simulink model "sendRecieve"  (R2016a)
settings: Solver=VariableStepAuto  StartTime=0.0  StopTime=10.0  RelTol=1e-3
libraries: instrumentlib x3
settings Model: Creator=Ori  LastModifiedBy=Ori

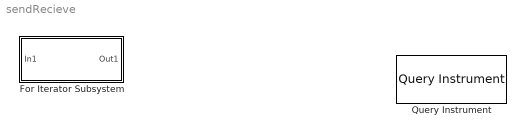
== system sendRecieve ==
  For Iterator Subsystem : Subsystem  TreatAsAtomicUnit=on
  Query Instrument : instrumentlib/Query Instrument  sampleTime=1  isWorkspaceObject=off  timeout=10  inputBufferSize=512  protocol=Serial  serialPort=COM1  baudRate=9600  gpibVendor=Advantech  boardIndex=0  primaryAddress=1  secondaryAddress=0  visaVendor=Agilent  visaSerialPort=0  chassisIndex=0  logicalAddress=0  tcpRemoteHost='127.0.0.1'  tcpRemotePort=4500  udpRemoteHost='127.0.0.1'  udpRemotePort=9090  visaTCPBoardIndex=0  visaTCPRemoteHost='127.0.0.1'  usbBoardIndex=0  usbManufID=0  usbModelCode=0  usbSerialNumber=0  initAction=None  initCommand='DATA:SOURCE CH1'  initFunction=get  queryCommand='curve?'  responseFormat=ASCII  asciiFormatting='%d,'  precision=8-bit integer  byteOrder=Little Endian  valuesToRead=1  removeBytes=off  afterOutputAction=Repeat query for new data  enableFrames=off  frameSize=1

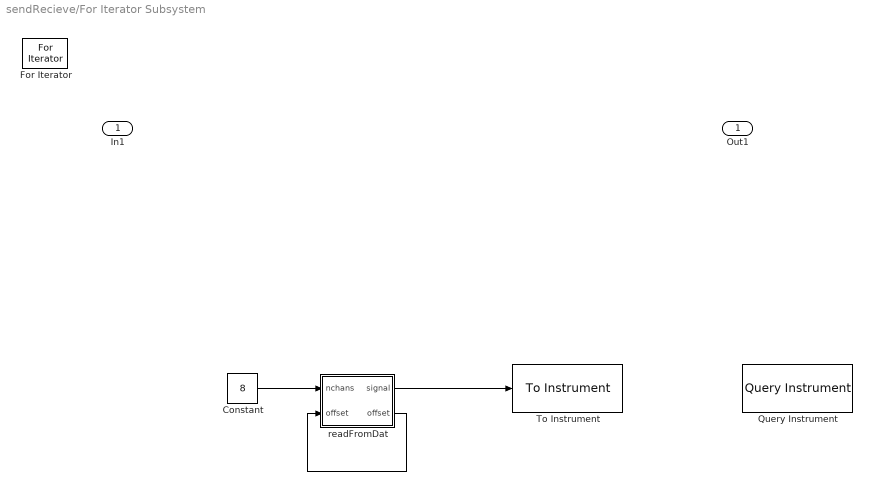
== system sendRecieve/For Iterator Subsystem ==
  In1 : Inport
  Constant : Constant  Value=8
  For Iterator : ForIterator
  Query Instrument : instrumentlib/Query Instrument  sampleTime=1  isWorkspaceObject=off  timeout=10  inputBufferSize=512  protocol=Serial  serialPort=COM1  baudRate=9600  gpibVendor=Advantech  boardIndex=0  primaryAddress=1  secondaryAddress=0  visaVendor=Agilent  visaSerialPort=0  chassisIndex=0  logicalAddress=0  tcpRemoteHost='127.0.0.1'  tcpRemotePort=4500  udpRemoteHost='127.0.0.1'  udpRemotePort=9090  visaTCPBoardIndex=0  visaTCPRemoteHost='127.0.0.1'  usbBoardIndex=0  usbManufID=0  usbModelCode=0  usbSerialNumber=0  initAction=None  initCommand='DATA:SOURCE CH1'  initFunction=get  queryCommand='curve?'  responseFormat=ASCII  asciiFormatting='%d,'  precision=8-bit integer  byteOrder=Little Endian  valuesToRead=1  removeBytes=off  afterOutputAction=Repeat query for new data  enableFrames=off  frameSize=1
  To Instrument : instrumentlib/To Instrument  sampleTime=-1  isWorkspaceObject=off  timeout=10  inputBufferSize=8192  protocol=Serial  serialPort=COM1  baudRate=9600  gpibVendor=Advantech  boardIndex=0  primaryAddress=1  secondaryAddress=0  visaVendor=Agilent  visaSerialPort=0  chassisIndex=0  logicalAddress=0  tcpRemoteHost='127.0.0.1'  tcpRemotePort=4500  udpRemoteHost='127.0.0.1'  udpRemotePort=9090  visaTCPBoardIndex=0  visaTCPRemoteHost='127.0.0.1'  usbBoardIndex=0  usbManufID=0  usbModelCode=0  usbSerialNumber=0  initAction=None  initCommand='DATA:SOURCE CH1'  initFunction=get  command=''  sendFormat=ASCII  asciiFormatting='%d'  precision=8-bit integer  byteOrder=Little Endian
  readFromDat : MATLAB Function  TreatAsAtomicUnit=on
  Out1 : Outport
  wires:
  Constant/1 -> readFromDat/1(nchans)
  readFromDat/1(signal) -> To Instrument/1
  readFromDat/2(offset) -> readFromDat/2("offset ")

== matlab function sendRecieve/For Iterator Subsystem/readFromDat ==
  data: nchans input; offset input; signal output; offset output
function [signal,offset] = fcn(nchans,offset)
%#codegen
if nargin == 1
    offset = 0;
end
fpath = []; % set fpath
files = dir(fullfile(fpath,'*.dat'));
idx = ~cellfun(@isempty,strfind({files.name},'temp_wh'));

fid = fopen(fullfile(fpath,files(idx).name));
fseek(fid, offset, 'bof');
signal = fread(fid,[nchans,1],'*int16');
offset = offset + 1;
